simulink model "UkladNieZeroweWarunkiJedenD"  (R2016a)
settings: Solver=ode45  StartTime=0.0  StopTime=10.0  MinStep=0.001  RelTol=1e-5
values from neighbouring files (symbols this model uses):
  A = [-100 0 0 ... (first row only)    [zad1.m]
  B = [1000 ... (first row only)    [zad1.m]
  C = [0 0 0.4]    [zad1.m]
  GDyskretne = acker(systemDyskretny.A',systemDyskretny.C',[exp(T*-14),exp(T*-28),exp(T*-36)])'    [zad1.m]
settings Model: Creator=student  LastModifiedBy=student

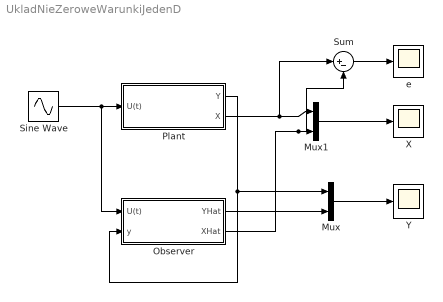
== system UkladNieZeroweWarunkiJedenD ==
  Mux : Mux  Inputs=2
  Mux1 : Mux  Inputs=2
  "Observer " : Subsystem
  Plant : Subsystem
  Sine Wave : Sin  SampleTime=0
  Sum : Sum  Inputs=|+-
  X : Scope
  Y : Scope
  e : Scope
  wires:
  Sine Wave/1 -> "Observer "/1(U(t)), Plant/1(U(t))
  Plant/1(Y) -> Mux/1, "Observer "/2("y ")
  "Observer "/1(YHat) -> Mux/2
  Plant/2(X) -> Sum/1, Mux1/1
  "Observer "/2(XHat) -> Sum/2, Mux1/2
  Mux1/1 -> X/1
  Mux/1 -> Y/1
  Sum/1 -> e/1

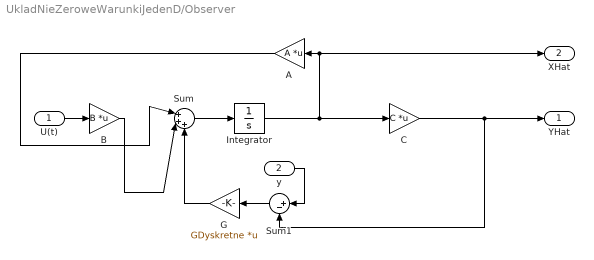
== system UkladNieZeroweWarunkiJedenD/Observer  ==
  U(t) : Inport
  "y " : Inport  Port=2
  A : Gain  Gain=A  Multiplication=Matrix(K*u)
  B : Gain  Gain=B  Multiplication=Matrix(K*u)
  C : Gain  Gain=C  Multiplication=Matrix(K*u)
  G : Gain  Gain=GDyskretne  Multiplication=Matrix(K*u)
  Integrator : Integrator  InitialCondition=[1 1 1]
  Sum : Sum  Inputs=|+++
  Sum1 : Sum  Inputs=|+-
  YHat : Outport
  XHat : Outport  Port=2
  wires:
  A/1 -> Sum/1
  U(t)/1 -> B/1
  Integrator/1 -> C/1, XHat/1, A/1
  C/1 -> Sum1/2, YHat/1
  B/1 -> Sum/2
  Sum/1 -> Integrator/1
  "y "/1 -> Sum1/1
  Sum1/1 -> G/1
  G/1 -> Sum/3

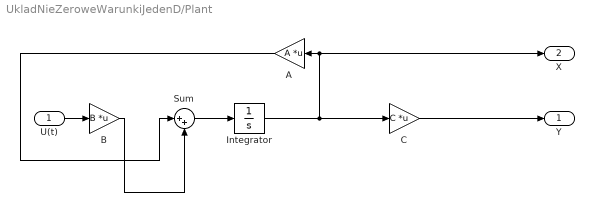
== system UkladNieZeroweWarunkiJedenD/Plant ==
  U(t) : Inport
  A : Gain  Gain=A  Multiplication=Matrix(K*u)
  B : Gain  Gain=B  Multiplication=Matrix(K*u)
  C : Gain  Gain=C  Multiplication=Matrix(K*u)
  Integrator : Integrator
  Sum : Sum  Inputs=|++
  Y : Outport
  X : Outport  Port=2
  wires:
  A/1 -> Sum/1
  U(t)/1 -> B/1
  Integrator/1 -> C/1, X/1, A/1
  C/1 -> Y/1
  B/1 -> Sum/2
  Sum/1 -> Integrator/1
